simulink model "Subsystem"  (R2020b)
settings: Solver=VariableStepAuto  StartTime=0.0  StopTime=10.0  RelTol=1e-3
values from neighbouring files (symbols this model uses):
  Kd = 6.98    [Variables.m]
  Ki = 12396450.71    [Variables.m]
  Kp = 18842.98    [Variables.m]
settings Model: DataDictionary=Data_Dictionary.sldd  Creator=samar  LastModifiedBy=samar
settings DataIOCC: SaveOutput=off  SaveTime=off

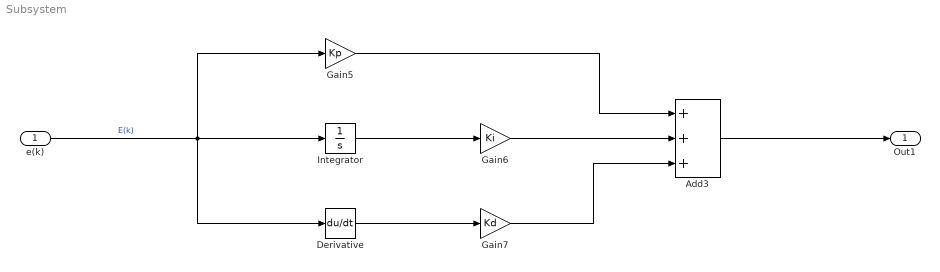
== system Subsystem ==
  e(k) : Inport  OutDataTypeStr=double  PortDimensions=1  SampleTime=0
  Add3 : Sum  Inputs=+++
  Derivative : Derivative
  Gain5 : Gain  Gain=Kp
  Gain6 : Gain  Gain=Ki
  Gain7 : Gain  Gain=Kd
  Integrator : Integrator
  Out1 : Outport  OutDataTypeStr=double  PortDimensions=1  SampleTime=0
  wires:
  Derivative/1 -> Gain7/1
  e(k)/1 -> Gain5/1, Integrator/1, Derivative/1  "E(k)"
  Gain5/1 -> Add3/1
  Integrator/1 -> Gain6/1
  Gain6/1 -> Add3/2
  Gain7/1 -> Add3/3
  Add3/1 -> Out1/1
